simulink model "SVPWM"  (R2022a)
settings: Solver=FixedStepDiscrete  StartTime=0.0  StopTime=0.1  FixedStep=1e-6  RelTol=1e-3
InitFcn:
  | f = 5000;
  | Ts = 1/f;
  | Vdc=48;
  | %m=sqrt(3)*311/Vdc;
  | m=0.8;
libraries: spsIGBTDiodeLib x6, spsSeriesRLCBranchLib x6, spsCurrentMeasurementLib x3, spsVoltageMeasurementLib x3, simulink x2, spsDCVoltageSourceLib x1, spspowerguiLib x1
settings Model: Creator=XieXW  LastModifiedBy=XieXW

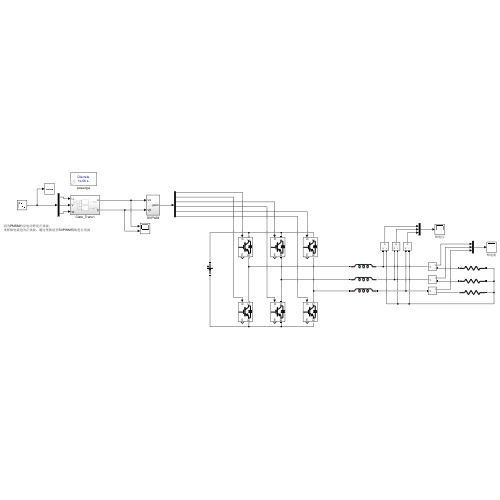
[thumbnail: Simulink's stored preview of the top-level diagram]
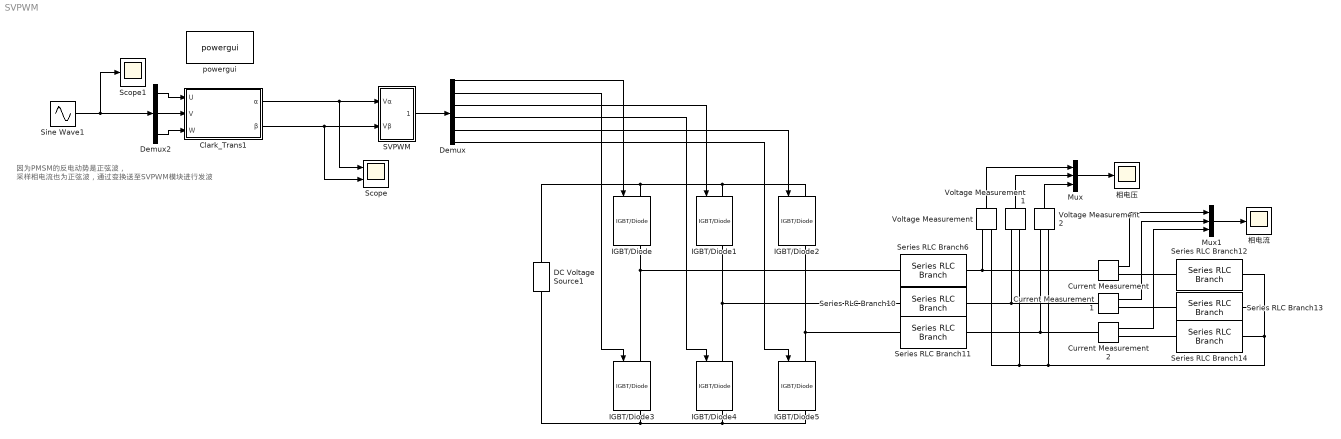
== system SVPWM ==
  note: 因为PMSM的反电动势是正弦波，
      | 采样相电流也为正弦波，通过变换送至SVPWM模块进行发波
  Clark_Trans1 : Subsystem
  Current Measurement : spsCurrentMeasurementLib/Current Measurement  PhasorSimulation=off  OutputType=Complex  PSBequivalent=0
  Current Measurement1 : spsCurrentMeasurementLib/Current Measurement  PhasorSimulation=off  OutputType=Complex  PSBequivalent=0
  Current Measurement2 : spsCurrentMeasurementLib/Current Measurement  PhasorSimulation=off  OutputType=Complex  PSBequivalent=0
  DC Voltage Source1 : spsDCVoltageSourceLib/DC Voltage Source  Amplitude=Vdc  Measurements=None
  Demux : Demux  Outputs=6
  Demux2 : Demux  Outputs=3
  IGBT/Diode{,1..5} (6 alike) : spsIGBTDiodeLib/IGBT//Diode  Ron=1e-3  Rs=1e5  Cs=inf  Measurements=on
  Mux : Mux  Inputs=3
  Mux1 : Mux  Inputs=3
  SVPWM : Subsystem
  Scope : Scope  NumInputPorts=2
  Scope1 : Scope
  Series RLC Branch10 : spsSeriesRLCBranchLib/Series RLC Branch  LConnTagsString=__new0  RConnTagsString=__new0  BranchType=L  Resistance=500  Inductance=0.01  SetiL0=off  InitialCurrent=0  Capacitance=0  Setx0=off  InitialVoltage=0  Measurements=None
  Series RLC Branch11 : spsSeriesRLCBranchLib/Series RLC Branch  LConnTagsString=__new0  RConnTagsString=__new0  BranchType=L  Resistance=500  Inductance=0.01  SetiL0=off  InitialCurrent=0  Capacitance=0  Setx0=off  InitialVoltage=0  Measurements=None
  Series RLC Branch12 : spsSeriesRLCBranchLib/Series RLC Branch  LConnTagsString=__new0  RConnTagsString=__new0  BranchType=R  Resistance=10  Inductance=0.005  SetiL0=off  InitialCurrent=0  Capacitance=0  Setx0=off  InitialVoltage=0  Measurements=None
  Series RLC Branch13 : spsSeriesRLCBranchLib/Series RLC Branch  LConnTagsString=__new0  RConnTagsString=__new0  BranchType=R  Resistance=10  Inductance=0.005  SetiL0=off  InitialCurrent=0  Capacitance=0  Setx0=off  InitialVoltage=0  Measurements=None
  Series RLC Branch14 : spsSeriesRLCBranchLib/Series RLC Branch  LConnTagsString=__new0  RConnTagsString=__new0  BranchType=R  Resistance=10  Inductance=0.005  SetiL0=off  InitialCurrent=0  Capacitance=0  Setx0=off  InitialVoltage=0  Measurements=None
  Series RLC Branch6 : spsSeriesRLCBranchLib/Series RLC Branch  LConnTagsString=__new0  RConnTagsString=__new0  BranchType=L  Resistance=500  Inductance=0.01  SetiL0=off  InitialCurrent=0  Capacitance=0  Setx0=off  InitialVoltage=0  Measurements=None
  Sine Wave1 : Sin  Amplitude=m  Frequency=50*pi*2  Phase=[0 -2*pi/3 2*pi/3]  SampleTime=0
  Voltage Measurement : spsVoltageMeasurementLib/Voltage Measurement  PhasorSimulation=off  OutputType=Complex  PSBequivalent=0
  Voltage Measurement1 : spsVoltageMeasurementLib/Voltage Measurement  PhasorSimulation=off  OutputType=Complex  PSBequivalent=0
  Voltage Measurement2 : spsVoltageMeasurementLib/Voltage Measurement  PhasorSimulation=off  OutputType=Complex  PSBequivalent=0
  powergui : spspowerguiLib/powergui  Priority=1  SimulationMode=Discrete  SampleTime=1e-6  frequency=60  Iterations=50  frequencyindice=0  Pbase=100e6  ErrMax=1e-4  UnitsV=kV  UnitsW=MW  buscounter=0  FunctionMessages=off  echomessages=off  EnableUseOfTLC=off  CurrentSourceSwitches=off  DisableSnubberDevices=off  DisableRonSwitches=off  DisableVfSwitches=off  DisplayEquations=off  AutomaticDiscreteSolvers=off  SolverType=Tustin/Backward Euler (TBE)  Interpol=off  ExternalGateDelay=off  methode=off  Ts=100  x0status=blocks  SPID=on  SwTol=0  HookPort=off  NonlinearTolerance=1e-4  nMaxIteration=100  ContinueOnMaxIteration=off  RestoreLinks=warning  ResistiveCurrentMeasurement=off  Frange=[0:2:500]  Ylog=off  Xlog=on  ShowGrid=off  save=off  variable=ZData  structure=0  ZoomFFT=off  StartTime=0.0  cycles=1  DisplayStyle=1  fundamental=60  FreqAxis=off  MaxFrequency=1000  frequencyindicesteady=1  RmsSteady=1  display=off
  相电压 : Scope
  相电流 : Scope
  wires:
  Demux2/2 -> Clark_Trans1/2(V)
  Demux2/1 -> Clark_Trans1/1(U)
  Demux2/3 -> Clark_Trans1/3(W)
  Clark_Trans1/1(α) -> Scope/1, SVPWM/1(Vα)
  Clark_Trans1/2(β) -> Scope/2, SVPWM/2(Vβ)
  SVPWM/1(pwm) -> Demux/1
  Demux/1 -> IGBT/Diode/1
  Demux/2 -> IGBT/Diode3/1
  Demux/3 -> IGBT/Diode1/1
  Demux/4 -> IGBT/Diode4/1
  Demux/5 -> IGBT/Diode2/1
  Demux/6 -> IGBT/Diode5/1
  Voltage Measurement/1 -> Mux/1
  Sine Wave1/1 -> Demux2/1, Scope1/1
  Mux/1 -> 相电压/1
  Voltage Measurement1/1 -> Mux/2
  Voltage Measurement2/1 -> Mux/3
  Current Measurement/1 -> Mux1/1
  Current Measurement1/1 -> Mux1/2
  Current Measurement2/1 -> Mux1/3
  Mux1/1 -> 相电流/1
  connections:
  DC Voltage Source1/RConn1 -- IGBT/Diode2/LConn1 -- IGBT/Diode1/LConn1 -- IGBT/Diode/LConn1
  DC Voltage Source1/LConn1 -- IGBT/Diode5/RConn1 -- IGBT/Diode4/RConn1 -- IGBT/Diode3/RConn1
  IGBT/Diode/RConn1 -- Series RLC Branch6/LConn1 -- IGBT/Diode3/LConn1
  IGBT/Diode1/RConn1 -- Series RLC Branch10/LConn1 -- IGBT/Diode4/LConn1
  IGBT/Diode2/RConn1 -- Series RLC Branch11/LConn1 -- IGBT/Diode5/LConn1
  Current Measurement/LConn1 -- Voltage Measurement/LConn1 -- Series RLC Branch6/RConn1
  Current Measurement1/RConn1 -- Series RLC Branch13/LConn1
  Current Measurement1/LConn1 -- Series RLC Branch10/RConn1 -- Voltage Measurement1/LConn1
  Current Measurement2/LConn1 -- Series RLC Branch11/RConn1 -- Voltage Measurement2/LConn1
  Series RLC Branch14/LConn1 -- Current Measurement2/RConn1
  Series RLC Branch12/RConn1 -- Voltage Measurement/LConn2 -- Voltage Measurement1/LConn2 -- Voltage Measurement2/LConn2 -- Series RLC Branch14/RConn1 -- Series RLC Branch13/RConn1
  Current Measurement/RConn1 -- Series RLC Branch12/LConn1

== system SVPWM/Clark_Trans1 ==
  U : Inport
  V : Inport  Port=2
  W : Inport  Port=3
  MATLAB Function : MATLAB Function  TreatAsAtomicUnit=on
  MATLAB Function1 : MATLAB Function  TreatAsAtomicUnit=on
  α : Outport
  β : Outport  Port=2
  wires:
  U/1 -> MATLAB Function/1(u)
  V/1 -> MATLAB Function1/1(v), MATLAB Function/2(v)
  W/1 -> MATLAB Function1/2(w), MATLAB Function/3(w)
  MATLAB Function/1(alpha) -> α/1
  MATLAB Function1/1(beta) -> β/1

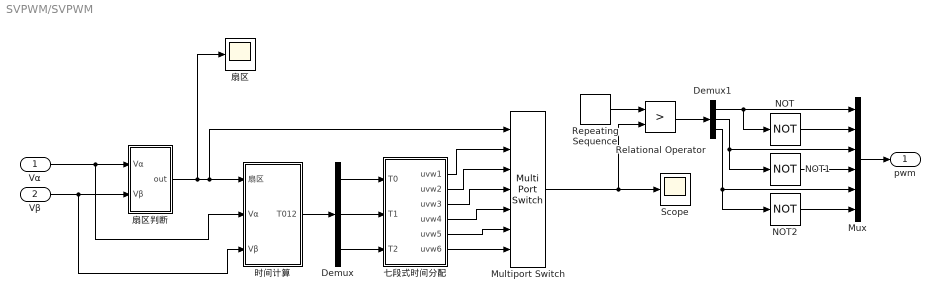
== system SVPWM/SVPWM ==
  Vα : Inport
  Vβ : Inport  Port=2
  Demux : Demux  Outputs=3
  Demux1 : Demux  Outputs=3
  Multiport Switch : MultiPortSwitch  Inputs=6  SaturateOnIntegerOverflow=off  InputSameDT=off
  Mux : Mux  Inputs=6
  NOT : Logic  Operator=NOT  IconShape=distinctive  AllPortsSameDT=off  OutDataTypeStr=boolean
  NOT1 : Logic  Operator=NOT  IconShape=distinctive  AllPortsSameDT=off  OutDataTypeStr=boolean
  NOT2 : Logic  Operator=NOT  IconShape=distinctive  AllPortsSameDT=off  OutDataTypeStr=boolean
  Relational Operator : RelationalOperator  Operator=>  OutDataTypeStr=boolean  RndMeth=Simplest  InputSameDT=off
  Repeating Sequence : simulink/Sources/Repeating Sequence  rep_seq_t=[0 Ts/2 Ts]  rep_seq_y=[0 1 0]
  Scope : Scope
  七段式时间分配 : Subsystem
  扇区 : Scope
  扇区判断 : Subsystem
  时间计算 : Subsystem
  pwm : Outport
  wires:
  七段式时间分配/6(uvw6) -> Multiport Switch/7
  Demux1/3 -> NOT2/1, Mux/5
  七段式时间分配/5(uvw5) -> Multiport Switch/6
  Demux1/2 -> NOT1/1, Mux/3
  Relational Operator/1 -> Demux1/1
  Demux/1 -> 七段式时间分配/1(T0)
  扇区判断/1(out) -> Multiport Switch/1, 时间计算/1(扇区), 扇区/1
  七段式时间分配/2(uvw2) -> Multiport Switch/3
  Vα/1 -> 时间计算/2(Vα), 扇区判断/1(Vα)
  Vβ/1 -> 时间计算/3(Vβ), 扇区判断/2(Vβ)
  七段式时间分配/1(uvw1) -> Multiport Switch/2
  时间计算/1(T012) -> Demux/1
  七段式时间分配/4(uvw4) -> Multiport Switch/5
  Demux/2 -> 七段式时间分配/2(T1)
  Multiport Switch/1 -> Relational Operator/2, Scope/1
  七段式时间分配/3(uvw3) -> Multiport Switch/4
  Demux/3 -> 七段式时间分配/3(T2)
  Repeating Sequence/1 -> Relational Operator/1
  Demux1/1 -> Mux/1, NOT/1
  NOT2/1 -> Mux/6
  NOT1/1 -> Mux/4
  NOT/1 -> Mux/2
  Mux/1 -> pwm/1

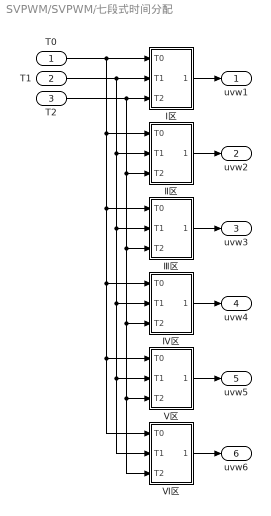
== system SVPWM/SVPWM/七段式时间分配 ==
  T0 : Inport
  T1 : Inport  Port=2
  T2 : Inport  Port=3
  Ⅰ区 : Subsystem
  Ⅱ区 : Subsystem
  Ⅲ区 : Subsystem
  Ⅳ区 : Subsystem
  Ⅴ区 : Subsystem
  Ⅵ区 : Subsystem
  uvw1 : Outport
  uvw2 : Outport  Port=2
  uvw3 : Outport  Port=3
  uvw4 : Outport  Port=4
  uvw5 : Outport  Port=5
  uvw6 : Outport  Port=6
  wires:
  Ⅱ区/1(uvw2) -> uvw2/1
  T1/1 -> Ⅵ区/2(T1), Ⅴ区/2(T1), Ⅳ区/2(T1), Ⅲ区/2(T1), Ⅱ区/2(T1), Ⅰ区/2(T1)
  Ⅰ区/1(uvw1) -> uvw1/1
  T2/1 -> Ⅵ区/3(T2), Ⅴ区/3(T2), Ⅳ区/3(T2), Ⅲ区/3(T2), Ⅱ区/3(T2), Ⅰ区/3(T2)
  Ⅳ区/1(uvw4) -> uvw4/1
  T0/1 -> Ⅱ区/1(T0), Ⅵ区/1(T0), Ⅴ区/1(T0), Ⅳ区/1(T0), Ⅲ区/1(T0), Ⅰ区/1(T0)
  Ⅵ区/1(uvw6) -> uvw6/1
  Ⅲ区/1(uvw3) -> uvw3/1
  Ⅴ区/1(uvw5) -> uvw5/1

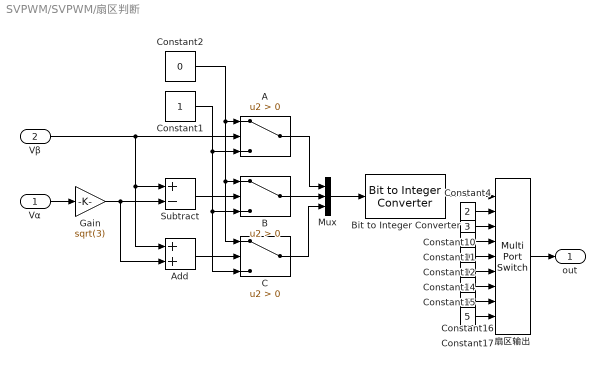
== system SVPWM/SVPWM/扇区判断 ==
  Vα : Inport
  Vβ : Inport  Port=2
  A : Switch  Criteria=u2 > Threshold  SaturateOnIntegerOverflow=off  InputSameDT=off
  Add : Sum
  B : Switch  Criteria=u2 > Threshold  SaturateOnIntegerOverflow=off  InputSameDT=off
  Bit to Integer Converter : simulink/Logic and Bit Operations/Bit to Integer Converter  nbits=3  bitOrder=MSB first  signedOutputValues=Unsigned  outDtype=Inherit via internal rule  outDtypeSigned=Inherit via internal rule
      settings: SourceProductBaseCode=SL
  C : Switch  Criteria=u2 > Threshold  SaturateOnIntegerOverflow=off  InputSameDT=off
  Constant1 : Constant
  Constant10 : Constant  Value=3
  Constant11 : Constant
  Constant12 : Constant  Value=0
  Constant14 : Constant  Value=0
  Constant15 : Constant  Value=4
  Constant16 : Constant  Value=6
  Constant17 : Constant  Value=5
  Constant2 : Constant  Value=0
  Constant4 : Constant  Value=2
  Gain : Gain  Gain=sqrt(3)
  Mux : Mux  Inputs=3
  Subtract : Sum  Inputs=+-
  扇区输出 : MultiPortSwitch  DataPortOrder=Zero-based contiguous  Inputs=8  zeroidx=on  SaturateOnIntegerOverflow=off  InputSameDT=off
  out : Outport
  wires:
  A/1 -> Mux/1
  Vβ/1 -> A/2, Add/1, Subtract/1
  Mux/1 -> Bit to Integer Converter/1
  Subtract/1 -> B/2
  B/1 -> Mux/2
  Constant2/1 -> C/1, B/1, A/1
  Gain/1 -> Add/2, Subtract/2
  Constant1/1 -> C/3, B/3, A/3
  C/1 -> Mux/3
  Add/1 -> C/2
  Vα/1 -> Gain/1
  扇区输出/1 -> out/1
  Bit to Integer Converter/1 -> 扇区输出/1
  Constant4/1 -> 扇区输出/2
  Constant10/1 -> 扇区输出/3
  Constant11/1 -> 扇区输出/4
  Constant12/1 -> 扇区输出/5
  Constant14/1 -> 扇区输出/6
  Constant15/1 -> 扇区输出/7
  Constant16/1 -> 扇区输出/8
  Constant17/1 -> 扇区输出/9

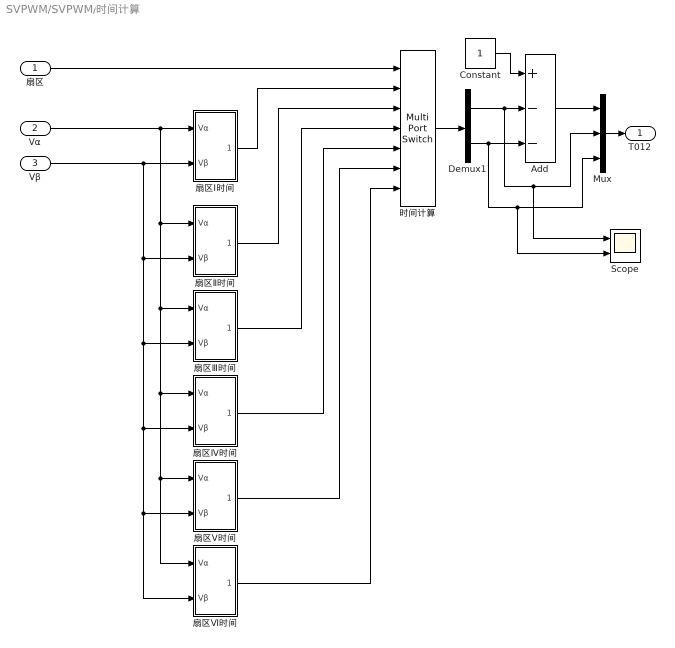
== system SVPWM/SVPWM/时间计算 ==
  扇区 : Inport
  Vα : Inport  Port=2
  Vβ : Inport  Port=3
  Add : Sum  Inputs=+--
  Constant : Constant
  Demux1 : Demux  Outputs=2
  Mux : Mux  Inputs=3
  Scope : Scope  NumInputPorts=2
  扇区Ⅰ时间 : Subsystem
  扇区Ⅱ时间 : Subsystem
  扇区Ⅲ时间 : Subsystem
  扇区Ⅳ时间 : Subsystem
  扇区Ⅴ时间 : Subsystem
  扇区Ⅵ时间 : Subsystem
  时间计算 : MultiPortSwitch  Inputs=6  SaturateOnIntegerOverflow=off  InputSameDT=off
  T012 : Outport
  wires:
  Vα/1 -> 扇区Ⅵ时间/1(Vα), 扇区Ⅴ时间/1(Vα), 扇区Ⅳ时间/1(Vα), 扇区Ⅲ时间/1(Vα), 扇区Ⅱ时间/1(Vα), 扇区Ⅰ时间/1(Vα)
  时间计算/1 -> Demux1/1
  Demux1/1 -> Scope/1, Mux/2, Add/2
  Add/1 -> Mux/1
  Demux1/2 -> Scope/2, Mux/3, Add/3
  Vβ/1 -> 扇区Ⅵ时间/2(Vβ), 扇区Ⅴ时间/2(Vβ), 扇区Ⅳ时间/2(Vβ), 扇区Ⅲ时间/2(Vβ), 扇区Ⅱ时间/2(Vβ), 扇区Ⅰ时间/2(Vβ)
  Constant/1 -> Add/1
  扇区Ⅰ时间/1(Tout1) -> 时间计算/2
  扇区Ⅴ时间/1(Tout5) -> 时间计算/6
  扇区Ⅳ时间/1(Tout4) -> 时间计算/5
  扇区Ⅱ时间/1(Tout2) -> 时间计算/3
  Mux/1 -> T012/1
  扇区Ⅵ时间/1(Tout6) -> 时间计算/7
  扇区Ⅲ时间/1(Tout3) -> 时间计算/4
  扇区/1 -> 时间计算/1

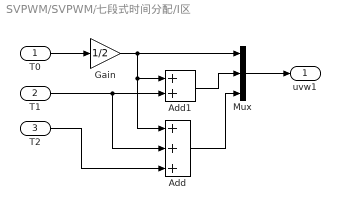
== system SVPWM/SVPWM/七段式时间分配/Ⅰ区 ==
  T0 : Inport
  T1 : Inport  Port=2
  T2 : Inport  Port=3
  Add : Sum  Inputs=+++
  Add1 : Sum
  Gain : Gain  Gain=1/2
  Mux : Mux  Inputs=3
  uvw1 : Outport
  wires:
  Add/1 -> Mux/3
  Gain/1 -> Add/1, Add1/1, Mux/1
  Add1/1 -> Mux/2
  T1/1 -> Add/2, Add1/2
  Mux/1 -> uvw1/1
  T2/1 -> Add/3
  T0/1 -> Gain/1

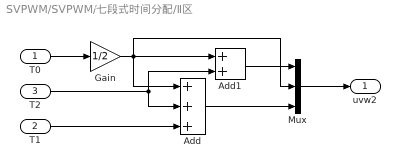
== system SVPWM/SVPWM/七段式时间分配/Ⅱ区 ==
  T0 : Inport
  T1 : Inport  Port=2
  T2 : Inport  Port=3
  Add : Sum  Inputs=+++
  Add1 : Sum
  Gain : Gain  Gain=1/2
  Mux : Mux  Inputs=3
  uvw2 : Outport
  wires:
  Mux/1 -> uvw2/1
  T0/1 -> Gain/1
  Gain/1 -> Add/1, Mux/2, Add1/1
  T2/1 -> Add/2, Add1/2
  Add1/1 -> Mux/1
  T1/1 -> Add/3
  Add/1 -> Mux/3

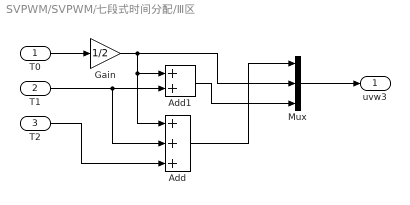
== system SVPWM/SVPWM/七段式时间分配/Ⅲ区 ==
  T0 : Inport
  T1 : Inport  Port=2
  T2 : Inport  Port=3
  Add : Sum  Inputs=+++
  Add1 : Sum
  Gain : Gain  Gain=1/2
  Mux : Mux  Inputs=3
  uvw3 : Outport
  wires:
  T0/1 -> Gain/1
  T2/1 -> Add/3
  Mux/1 -> uvw3/1
  T1/1 -> Add1/2, Add/2
  Gain/1 -> Mux/2, Add1/1, Add/1
  Add/1 -> Mux/1
  Add1/1 -> Mux/3

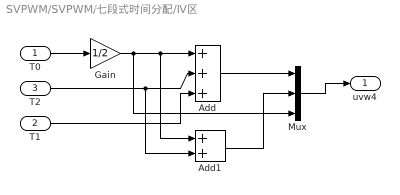
== system SVPWM/SVPWM/七段式时间分配/Ⅳ区 ==
  T0 : Inport
  T1 : Inport  Port=2
  T2 : Inport  Port=3
  Add : Sum  Inputs=+++
  Add1 : Sum
  Gain : Gain  Gain=1/2
  Mux : Mux  Inputs=3
  uvw4 : Outport
  wires:
  Gain/1 -> Add/1, Add1/1, Mux/3
  T0/1 -> Gain/1
  Mux/1 -> uvw4/1
  T2/1 -> Add1/2, Add/2
  T1/1 -> Add/3
  Add/1 -> Mux/1
  Add1/1 -> Mux/2

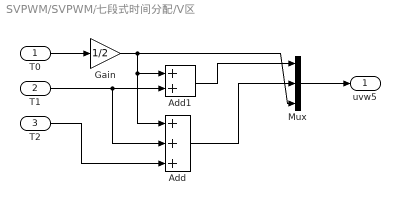
== system SVPWM/SVPWM/七段式时间分配/Ⅴ区 ==
  T0 : Inport
  T1 : Inport  Port=2
  T2 : Inport  Port=3
  Add : Sum  Inputs=+++
  Add1 : Sum
  Gain : Gain  Gain=1/2
  Mux : Mux  Inputs=3
  uvw5 : Outport
  wires:
  Gain/1 -> Add/1, Add1/1, Mux/3
  T1/1 -> Add/2, Add1/2
  Mux/1 -> uvw5/1
  T2/1 -> Add/3
  T0/1 -> Gain/1
  Add/1 -> Mux/2
  Add1/1 -> Mux/1

== system SVPWM/SVPWM/七段式时间分配/Ⅵ区 ==
  T0 : Inport
  T1 : Inport  Port=2
  T2 : Inport  Port=3
  Add : Sum  Inputs=+++
  Add1 : Sum
  Gain : Gain  Gain=1/2
  Mux : Mux  Inputs=3
  uvw6 : Outport
  wires:
  Mux/1 -> uvw6/1
  T0/1 -> Gain/1
  Gain/1 -> Add/1, Add1/2, Mux/1
  T2/1 -> Add/2, Add1/1
  T1/1 -> Add/3
  Add/1 -> Mux/2
  Add1/1 -> Mux/3

== system SVPWM/SVPWM/时间计算/扇区Ⅰ时间 ==
  Vα : Inport
  Vβ : Inport  Port=2
  Gain : Gain  Gain=1/2
  Mux : Mux  Inputs=2
  Subtract : Sum  Inputs=+-
  sqrt(3)/2 : Gain  Gain=sqrt(3)/2
  Tout1 : Outport
  wires:
  Gain/1 -> Subtract/2
  Vβ/1 -> Mux/2, Gain/1
  Subtract/1 -> Mux/1
  Mux/1 -> Tout1/1
  sqrt(3)/2/1 -> Subtract/1
  Vα/1 -> sqrt(3)/2/1

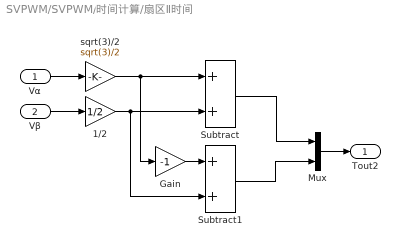
== system SVPWM/SVPWM/时间计算/扇区Ⅱ时间 ==
  Vα : Inport
  Vβ : Inport  Port=2
  1/2 : Gain  Gain=1/2
  Gain : Gain  Gain=-1
  Mux : Mux  Inputs=2
  Subtract : Sum
  Subtract1 : Sum
  sqrt(3)/2 : Gain  Gain=sqrt(3)/2
  Tout2 : Outport
  wires:
  Vα/1 -> sqrt(3)/2/1
  Mux/1 -> Tout2/1
  Subtract/1 -> Mux/1
  Vβ/1 -> 1/2/1
  1/2/1 -> Subtract1/2, Subtract/2
  sqrt(3)/2/1 -> Gain/1, Subtract/1
  Subtract1/1 -> Mux/2
  Gain/1 -> Subtract1/1

== system SVPWM/SVPWM/时间计算/扇区Ⅲ时间 ==
  Vα : Inport
  Vβ : Inport  Port=2
  1/2 : Gain  Gain=1/2
  Gain : Gain  Gain=-1
  Mux : Mux  Inputs=2
  Subtract1 : Sum
  sqrt(3)/2 : Gain  Gain=sqrt(3)/2
  Tout3 : Outport
  wires:
  Vβ/1 -> Mux/1, 1/2/1
  Mux/1 -> Tout3/1
  Vα/1 -> sqrt(3)/2/1
  sqrt(3)/2/1 -> Subtract1/1
  1/2/1 -> Subtract1/2
  Subtract1/1 -> Gain/1
  Gain/1 -> Mux/2

== system SVPWM/SVPWM/时间计算/扇区Ⅳ时间 ==
  Vα : Inport
  Vβ : Inport  Port=2
  -sqrt(3)/2 : Gain  Gain=-sqrt(3)/2
  1/2 : Gain  Gain=1/2
  Gain : Gain  Gain=-1
  Mux : Mux  Inputs=2
  Subtract : Sum
  Tout4 : Outport
  wires:
  Vα/1 -> -sqrt(3)/2/1
  Mux/1 -> Tout4/1
  Vβ/1 -> Gain/1, 1/2/1
  Gain/1 -> Mux/2
  1/2/1 -> Subtract/2
  -sqrt(3)/2/1 -> Subtract/1
  Subtract/1 -> Mux/1

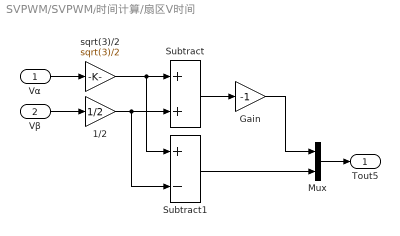
== system SVPWM/SVPWM/时间计算/扇区Ⅴ时间 ==
  Vα : Inport
  Vβ : Inport  Port=2
  1/2 : Gain  Gain=1/2
  Gain : Gain  Gain=-1
  Mux : Mux  Inputs=2
  Subtract : Sum
  Subtract1 : Sum  Inputs=+-
  sqrt(3)/2 : Gain  Gain=sqrt(3)/2
  Tout5 : Outport
  wires:
  1/2/1 -> Subtract1/2, Subtract/2
  Vβ/1 -> 1/2/1
  Mux/1 -> Tout5/1
  Vα/1 -> sqrt(3)/2/1
  sqrt(3)/2/1 -> Subtract1/1, Subtract/1
  Subtract/1 -> Gain/1
  Gain/1 -> Mux/1
  Subtract1/1 -> Mux/2

== system SVPWM/SVPWM/时间计算/扇区Ⅵ时间 ==
  Vα : Inport
  Vβ : Inport  Port=2
  1/2 : Gain  Gain=1/2
  Gain : Gain  Gain=-1
  Mux : Mux  Inputs=2
  Subtract1 : Sum
  sqrt(3)/2 : Gain  Gain=sqrt(3)/2
  Tout6 : Outport
  wires:
  Vα/1 -> sqrt(3)/2/1
  sqrt(3)/2/1 -> Subtract1/1
  Mux/1 -> Tout6/1
  Vβ/1 -> Gain/1, 1/2/1
  1/2/1 -> Subtract1/2
  Subtract1/1 -> Mux/2
  Gain/1 -> Mux/1

== matlab function SVPWM/Clark_Trans1/MATLAB Function1 ==
  data: beta output; v input; w input
function beta = fcn(v,w)

beta = (2/3)*((sqrt(3)/2)*v+(-sqrt(3)/2)*w);

== matlab function SVPWM/Clark_Trans1/MATLAB Function ==
  data: u input; alpha output; v input; w input
function alpha = fcn(u,v,w)

alpha = (2/3)*(u+(-1/2)*v+(-1/2)*w);
